simulink model "Hinf_GS_Control"  (Simulink 7.7)
settings: Solver=ode23tb  StartTime=0.0  StopTime=450  FixedStep=0.1  RelTol=1e-3
values from neighbouring files (symbols this model uses):
  Ac1 = K_1(1:ns,1:ns)    [example13_4.m]
  Ac2 = K_2(1:ns,1:ns)    [example13_4.m]
  Bc1 = K_1(1:ns,ns+1:ns+ni)    [example13_4.m]
  Bc2 = K_2(1:ns,ns+1:ns+ni)    [example13_4.m]
  Cc1 = K_1(ns+1:ns+no,1:ns)    [example13_4.m]
  Cc2 = K_2(ns+1:ns+no,1:ns)    [example13_4.m]
  G0 = 0.02    [plant_parameters.m]
  H0 = 1.0    (= 1)    [alpha_eval.m]    (also in plant_parameters.m)
  k = L*Pr/(ag*kp*Hr^2)    (= 4.67710019788)    [plant_parameters.m]
  Ts = 3    [example13_4.m]    (also in plant_parameters.m)
settings Model: Creator=ts_slavov  LastModifiedBy=Petko Petkov
settings OptimizationCC: InitFltsAndDblsToZero=on
settings DebuggingCC: SaveWithParameterizedLinksMsg=none  MultiTaskCondExecSysMsg=none  StrictBusMsg=Warning
settings RTWCC: IncludeERTFirstTime=on

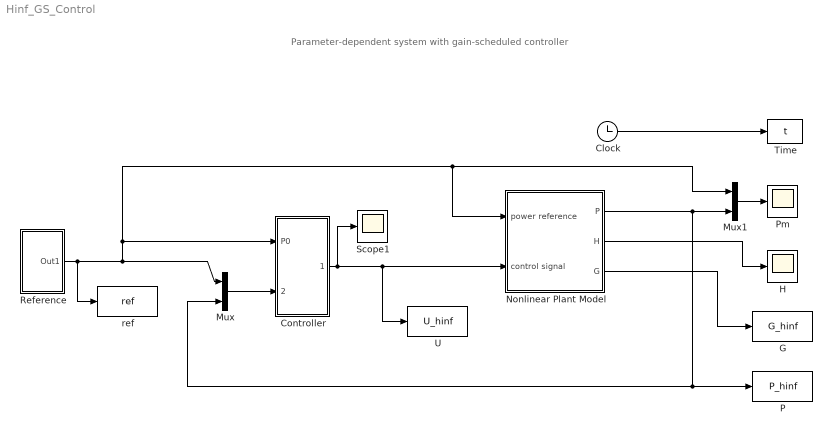
== system Hinf_GS_Control ==
  note: Parameter-dependent system with gain-scheduled controller
  Clock : Clock
  Controller : Subsystem
  G : ToWorkspace  VariableName=G_hinf  SampleTime=-1  SaveFormat=Structure With Time
  H : Scope
      settings: YMin=0.7973  YMax=0.79738  SaveName=ScopeData3
  Mux : Mux  Inputs=2
  Mux1 : Mux  Inputs=2
  Nonlinear Plant Model : Subsystem
  P : ToWorkspace  VariableName=P_hinf  SampleTime=-1  SaveFormat=Structure With Time
  Pm : Scope
      settings: YMin=0.7973  YMax=0.79738
  Reference : Subsystem
  Scope1 : Scope
      settings: YMin=0.163  YMax=0.179
  Time : ToWorkspace  VariableName=t  SampleTime=-1  SaveFormat=Array
  U : ToWorkspace  VariableName=U_hinf  SampleTime=-1  SaveFormat=Structure With Time
  ref : ToWorkspace  VariableName=ref  SampleTime=-1  SaveFormat=Structure With Time
  wires:
  Nonlinear Plant Model/1(P) -> P/1, Mux/2, Mux1/2
  Controller/1(Control) -> Scope1/1, Nonlinear Plant Model/2(control signal), U/1
  Reference/1(Out1) -> Mux/1, Controller/1(P0), Nonlinear Plant Model/1(power reference), Mux1/1, ref/1
  Nonlinear Plant Model/3(G) -> G/1
  Mux/1 -> Controller/2(error)
  Nonlinear Plant Model/2(H) -> H/1
  Clock/1 -> Time/1
  Mux1/1 -> Pm/1

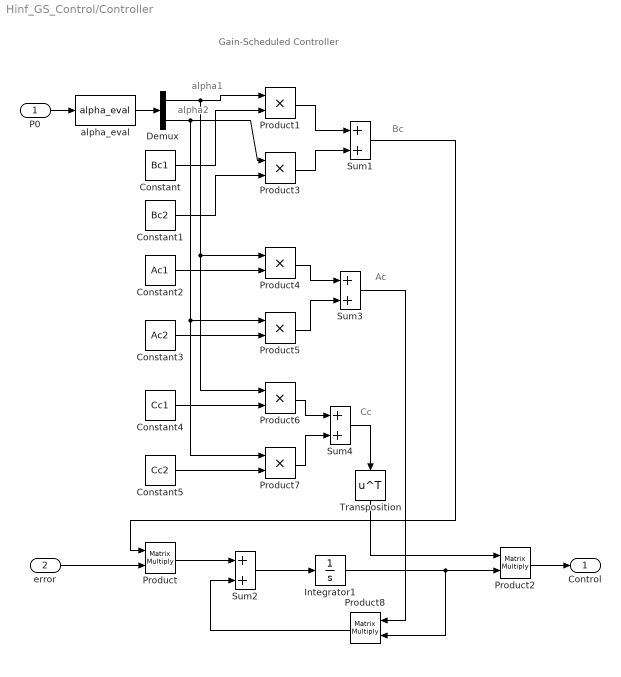
== system Hinf_GS_Control/Controller ==
  note: Bc
  note: alpha1
  note: alpha2
  note: Ac
  note: Cc
  note: Gain-Scheduled Controller
  P0 : Inport
  error : Inport  Port=2
  Constant : Constant  Value=Bc1
  Constant1 : Constant  Value=Bc2
  Constant2 : Constant  Value=Ac1
  Constant3 : Constant  Value=Ac2
  Constant4 : Constant  Value=Cc1
  Constant5 : Constant  Value=Cc2
  Demux : Demux  Outputs=2
  Integrator1 : Integrator
  Product : Product  Multiplication=Matrix(*)  RndMeth=Zero
  Product{1,3..7} (6 alike) : Product  RndMeth=Zero
  Product2 : Product  Multiplication=Matrix(*)  RndMeth=Zero
  Product8 : Product  Multiplication=Matrix(*)  RndMeth=Zero
  Sum{1..4} (4 alike) : Sum
  Transposition : Math  Operator=transpose  SaturateOnIntegerOverflow=on
  alpha_eval : MATLABFcn  MATLABFcn=alpha_eval  OutputDimensions=2  Output1D=off
  Control : Outport
  wires:
  Sum2/1 -> Integrator1/1
  Integrator1/1 -> Product2/2, Product8/2
  Product8/1 -> Sum2/2
  Product/1 -> Sum2/1
  P0/1 -> alpha_eval/1
  Product2/1 -> Control/1
  alpha_eval/1 -> Demux/1
  Demux/1 -> Product1/1, Product4/1, Product6/1
  Constant/1 -> Product1/2
  Demux/2 -> Product3/1, Product5/1, Product7/1
  Constant1/1 -> Product3/2
  Product1/1 -> Sum1/1
  Product3/1 -> Sum1/2
  Sum1/1 -> Product/1
  Constant2/1 -> Product4/2
  Constant3/1 -> Product5/2
  Product4/1 -> Sum3/1
  Product5/1 -> Sum3/2
  Sum3/1 -> Product8/1
  Constant4/1 -> Product6/2
  Constant5/1 -> Product7/2
  Product6/1 -> Sum4/1
  Product7/1 -> Sum4/2
  error/1 -> Product/2
  Sum4/1 -> Transposition/1
  Transposition/1 -> Product2/1

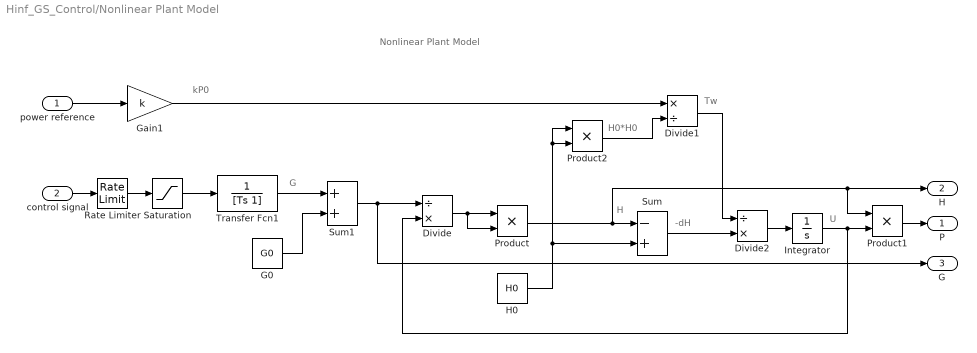
== system Hinf_GS_Control/Nonlinear Plant Model ==
  note: G
  note: U
  note: H
  note: -dH
  note: Nonlinear Plant Model
  note: Tw
  note: H0*H0
  note: kP0
  power reference : Inport
  control signal : Inport  Port=2
  Divide : Product  Inputs=/*
  Divide1 : Product  Inputs=*/
  Divide2 : Product  Inputs=/*
  G0 : Constant  Value=G0
  Gain1 : Gain  Gain=k
  H0 : Constant  Value=H0
  Integrator : Integrator  InitialCondition=1*0
  Product : Product  RndMeth=Zero
  Product1 : Product  RndMeth=Zero
  Product2 : Product  RndMeth=Zero
  Rate Limiter : RateLimiter  RisingSlewLimit=1/15  FallingSlewLimit=-1/15  SampleTimeMode=inherited
  Saturation : Saturate  UpperLimit=1  LowerLimit=0
  Sum : Sum  Inputs=-+
  Sum1 : Sum
  Transfer Fcn1 : TransferFcn  Denominator=[Ts 1]
  P : Outport
  H : Outport  Port=2
  G : Outport  Port=3
  wires:
  Divide/1 -> Product/1, Product/2
  Product/1 -> Sum/1, H/1, Product1/1
  H0/1 -> Sum/2, Product2/1, Product2/2
  Integrator/1 -> Product1/2, Divide/2
  Divide2/1 -> Integrator/1
  Product1/1 -> P/1
  Saturation/1 -> Transfer Fcn1/1
  control signal/1 -> Rate Limiter/1
  Rate Limiter/1 -> Saturation/1
  power reference/1 -> Gain1/1
  Gain1/1 -> Divide1/1
  Product2/1 -> Divide1/2
  Sum/1 -> Divide2/2
  Divide1/1 -> Divide2/1
  Transfer Fcn1/1 -> Sum1/1
  G0/1 -> Sum1/2
  Sum1/1 -> Divide/1, G/1

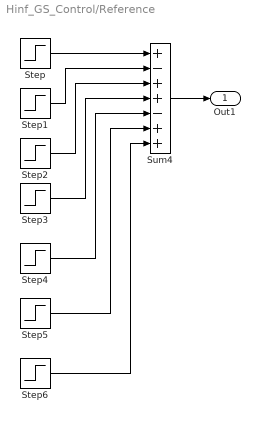
== system Hinf_GS_Control/Reference ==
  Step : Step  Time=0  After=0.8  SampleTime=0
  Step1 : Step  Time=60  After=0.3  SampleTime=0
  Step2 : Step  Time=120  After=-0.2  SampleTime=0
  Step3 : Step  Time=180  After=0.6  SampleTime=0
  Step4 : Step  Time=240  After=0.2  SampleTime=0
  Step5 : Step  Time=300  After=-0.3  SampleTime=0
  Step6 : Step  Time=360  After=0.4  SampleTime=0
  Sum4 : Sum  Inputs=+-++-++
  Out1 : Outport
  wires:
  Step/1 -> Sum4/1
  Step1/1 -> Sum4/2
  Step2/1 -> Sum4/3
  Step3/1 -> Sum4/4
  Step4/1 -> Sum4/5
  Step5/1 -> Sum4/6
  Step6/1 -> Sum4/7
  Sum4/1 -> Out1/1
